simulink model "Feedforward"  (R2022a)
settings: Solver=VariableStepAuto  StartTime=0.0  StopTime=1000  RelTol=1e-3
undefined symbols (not defined in the file): C, k, k1, k2, k3, keta
libraries: slpidlib x1
settings Model: Creator=Anca Lombrea  LastModifiedBy=Anca Lombrea

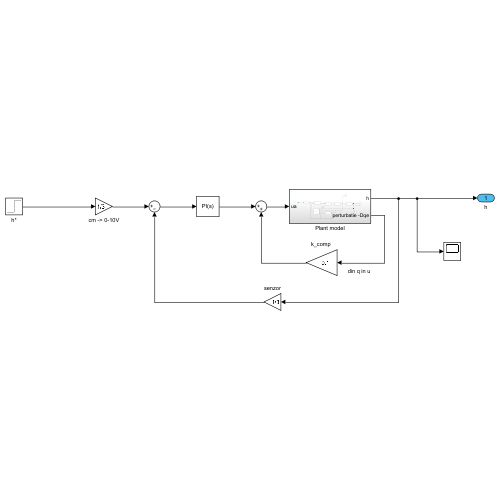
[thumbnail: Simulink's stored preview of the top-level diagram]
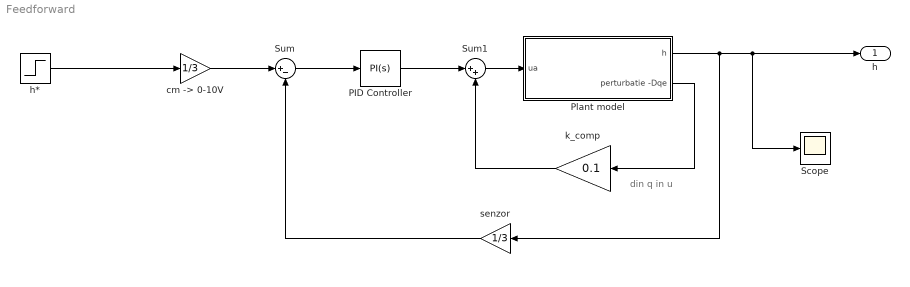
== system Feedforward ==
  note: din q in u
  PID Controller : slpidlib/PID Controller  Controller=PI  Form=Parallel  TimeDomain=Continuous-time  UseExternalTs=off  SampleTime=-1  IntegratorMethod=Forward Euler  FilterMethod=Forward Euler  ControllerParametersSource=internal  P=1.648  I=0.007925  UseKiTs=off  D=0  N=100  UseFilter=on  TunerSelectOption=Transfer Function Based (PID Tuner App)  InitialConditionSource=internal  InitialConditionForIntegrator=5.7  InitialConditionForFilter=0  DifferentiatorICPrevScaledInput=0  ExternalReset=none  TrackingMode=off  Kt=1  LimitOutput=off  SatLimitsSource=internal  UpperSaturationLimit=inf  LowerSaturationLimit=-inf  LinearizeAsGain=on  AntiWindupMode=none  Kb=1  POutMin=[]  POutMax=[]  IOutMin=[]  IOutMax=[]  DOutMin=[]  DOutMax=[]  NOutMin=[]  NOutMax=[]  SumOutMin=[]  SumOutMax=[]  SaturationOutMin=[]  SaturationOutMax=[]  PParamMin=[]  PParamMax=[]  IParamMin=[]  IParamMax=[]  DParamMin=[]  DParamMax=[]  NParamMin=[]  NParamMax=[]  KbParamMin=[]  KbParamMax=[]  KtParamMin=[]  KtParamMax=[]  KbOutMin=[]  KbOutMax=[]  KtOutMin=[]  KtOutMax=[]  IntegratorOutMin=[]  IntegratorOutMax=[]  FilterOutMin=[]  FilterOutMax=[]  SumI1OutMin=[]  SumI1OutMax=[]  SumI2OutMin=[]  SumI2OutMax=[]  SumI3OutMin=[]  SumI3OutMax=[]  SumI4OutMin=[]  SumI4OutMax=[]  SumDOutMin=[]  SumDOutMax=[]  DifferentiatorOutMin=[]  DifferentiatorOutMax=[]  FilterDiffOutCoefMin=[]  FilterDiffOutCoefMax=[]  ReciprocalOutMin=[]  ReciprocalOutMax=[]  SumDenOutMin=[]  SumDenOutMax=[]  SumNumOutMin=[]  SumNumOutMax=[]  DivideOutMin=[]  DivideOutMax=[]  UdiffTsProdOutMin=[]  UdiffTsProdOutMax=[]  NTsProdOutMin=[]  NTsProdOutMax=[]  UintegralTsProdOutMin=[]  UintegralTsProdOutMax=[]  UngainTsProdOutMin=[]  UngainTsProdOutMax=[]  IntegratorContinuousStateAttributes=''  IntegratorStateMustResolveToSignalObject=off  IntegratorRTWStateStorageClass=Auto  FilterContinuousStateAttributes=''  FilterStateMustResolveToSignalObject=off  FilterRTWStateStorageClass=Auto  ParallelPVariant=InternalParameters  IdealPVariant=Disabled  IVariant=InternalParameters  DVariant=Disabled  IntegratorVariant=Continuous  SatVariant=Disabled  AWVariant=Passthrough  PCopyVariant=Disabled  TRVariant=Disabled  FdbkBlocksVariant=Forward  IdealPFdbkVariant=Disabled  SatFdbkVariant=Disabled  DerivativeFilterVariant=Disabled  NVariant=Disabled  NCopyVariant=Disabled_SignalSpec  FilterICVariant=Disabled  IntegratorICVariant=InternalICs  ExternalResetVariant=Disabled  TRSumVariant=Passthrough  SumFdbkVariant=Disabled  SumVariant=Sum_PI  TsampFilterVariant=InternalTs  TsampNgainVariant=Passthrough  TsampIntegralVariant=Passthrough  ExternalSaturationOutDataTypeStr=Inherit: Same as second input  aMode=0
  Plant model : Subsystem
  Scope : Scope
  Sum : Sum  Inputs=|+-
  Sum1 : Sum  Inputs=|++
  "cm -> 0-10V" : Gain  Gain=1/3
  h* : Step  Time=0  After=20.87  SampleTime=0.01
  "k_comp " : Gain  Gain=0.1
  senzor : Gain  Gain=1/3
  h : Outport
  wires:
  senzor/1 -> Sum/2
  Sum/1 -> PID Controller/1
  Plant model/2(perturbatie -Dqe) -> "k_comp "/1
  h*/1 -> "cm -> 0-10V"/1
  Sum1/1 -> Plant model/1(ua)
  Plant model/1(h) -> senzor/1, Scope/1, h/1
  PID Controller/1 -> Sum1/1
  "cm -> 0-10V"/1 -> Sum/1
  "k_comp "/1 -> Sum1/2

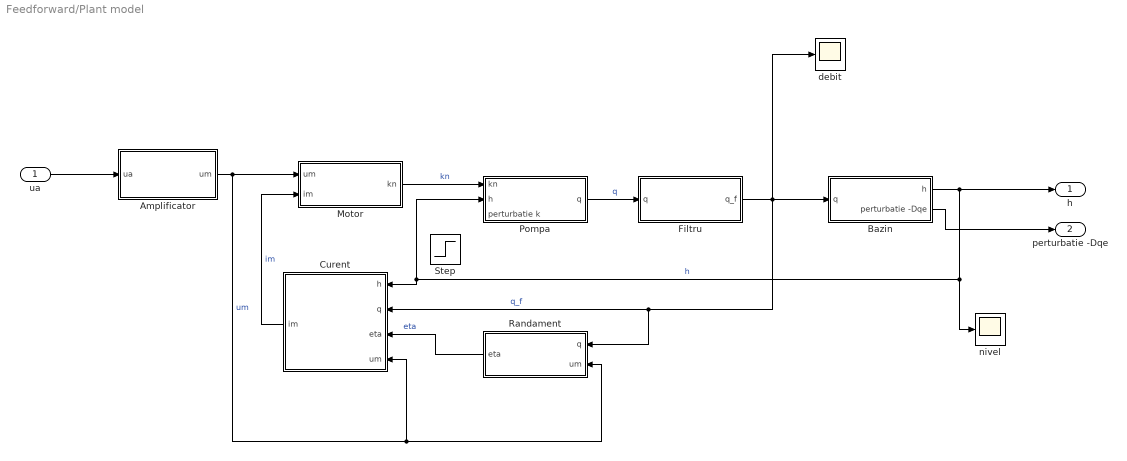
== system Feedforward/Plant model ==
  ua : Inport
  Amplificator : Subsystem
  Bazin : Subsystem
  Curent : Subsystem
  Filtru : Subsystem
  Motor : Subsystem
  Pompa : Subsystem
  Randament : Subsystem
  Step : Step  Time=250  Before=0.035  After=0.045  SampleTime=0
  debit : Scope
  nivel : Scope
  h : Outport
  perturbatie -Dqe : Outport  Port=2
  wires:
  Pompa/1("\tq") -> Filtru/1(q)  "q"
  Motor/1(kn) -> Pompa/1(kn)  "kn"
  Filtru/1(q_f) -> debit/1, Curent/2(q), Randament/1("\tq"), Bazin/1("\tq")  "q_f"
  ua/1 -> Amplificator/1(ua)
  Amplificator/1(um) -> Curent/4(um), Randament/2(um), Motor/1(um)  "um"
  Randament/1(eta) -> Curent/3(eta)  "eta"
  Bazin/1(h) -> nivel/1, Curent/1(h), Pompa/2(h), h/1  "h"
  Curent/1(im) -> Motor/2(im)  "im"
  Bazin/2(perturbatie -Dqe) -> perturbatie -Dqe/1

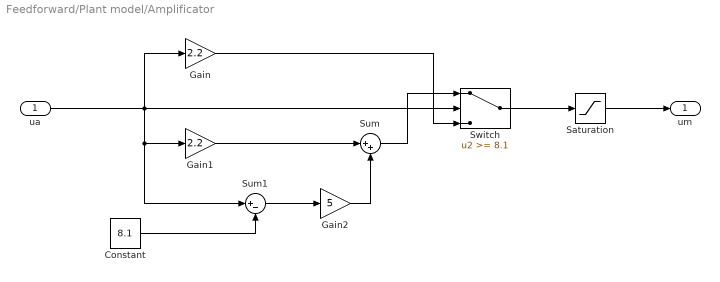
== system Feedforward/Plant model/Amplificator ==
  ua : Inport
  Constant : Constant  Value=8.1
  Gain : Gain  Gain=2.2
  Gain1 : Gain  Gain=2.2
  Gain2 : Gain  Gain=5
  Saturation : Saturate  UpperLimit=22  LowerLimit=0
  Sum : Sum  Inputs=|++
  Sum1 : Sum  Inputs=|+-
  Switch : Switch  Threshold=8.1  SaturateOnIntegerOverflow=off  InputSameDT=off
  um : Outport
  wires:
  Switch/1 -> Saturation/1
  Gain/1 -> Switch/3
  ua/1 -> Gain/1, Switch/2, Sum1/1, Gain1/1
  Gain2/1 -> Sum/2
  Constant/1 -> Sum1/2
  Sum/1 -> Switch/1
  Saturation/1 -> um/1
  Sum1/1 -> Gain2/1
  Gain1/1 -> Sum/1

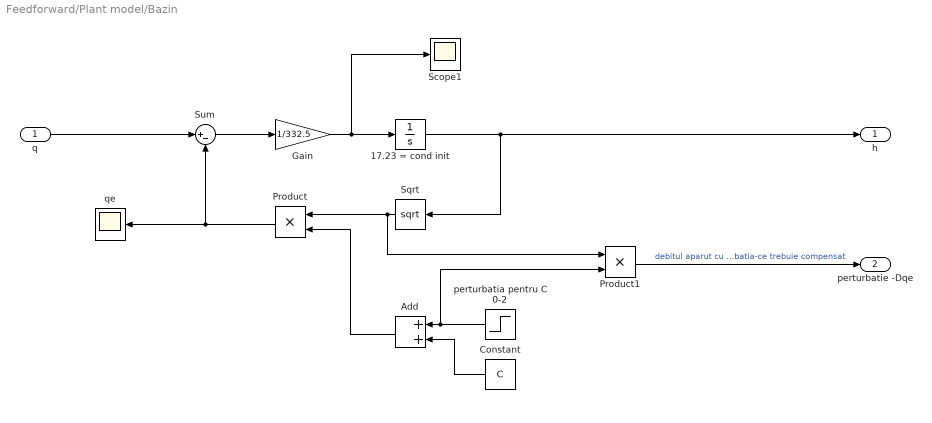
== system Feedforward/Plant model/Bazin ==
  "\tq" : Inport
  17.23 = cond init : Integrator  InitialCondition=17.23
  Add : Sum
  Constant : Constant  Value=C
  Gain : Gain  Gain=1/332.5
  Product : Product
  Product1 : Product
  Scope1 : Scope
  Sqrt : Sqrt
  Sum : Sum  Inputs=|+-
  "perturbatia pentru C 0-2 " : Step  Time=250  After=2  SampleTime=0
  qe : Scope
  h : Outport
  perturbatie -Dqe : Outport  Port=2
  wires:
  Sqrt/1 -> Product1/1, Product/1
  Product/1 -> qe/1, Sum/2
  "\tq"/1 -> Sum/1
  Sum/1 -> Gain/1
  17.23 = cond init/1 -> Sqrt/1, h/1
  Gain/1 -> 17.23 = cond init/1, Scope1/1
  "perturbatia pentru C 0-2 "/1 -> Product1/2, Add/1
  Constant/1 -> Add/2
  Add/1 -> Product/2
  Product1/1 -> perturbatie -Dqe/1  "debitul aparut cu perturbatia-ce trebuie compensat"

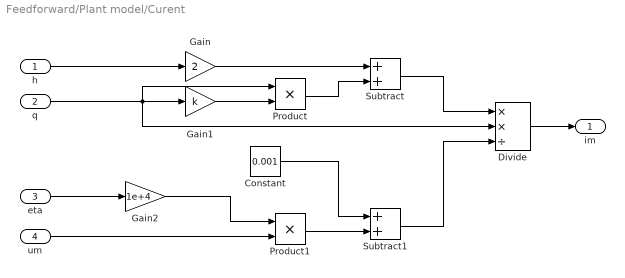
== system Feedforward/Plant model/Curent ==
  h : Inport
  q : Inport  Port=2
  eta : Inport  Port=3
  um : Inport  Port=4
  Constant : Constant  Value=0.001
  Divide : Product  Inputs=**/
  Gain : Gain  Gain=2
  Gain1 : Gain  Gain=k
  Gain2 : Gain  Gain=1e+4
  Product : Product
  Product1 : Product
  Subtract : Sum
  Subtract1 : Sum
  im : Outport
  wires:
  h/1 -> Gain/1
  Gain/1 -> Subtract/1
  q/1 -> Divide/2, Gain1/1, Product/1
  Gain1/1 -> Product/2
  Product/1 -> Subtract/2
  Subtract/1 -> Divide/1
  eta/1 -> Gain2/1
  Gain2/1 -> Product1/1
  um/1 -> Product1/2
  Product1/1 -> Subtract1/2
  Constant/1 -> Subtract1/1
  Subtract1/1 -> Divide/3
  Divide/1 -> im/1

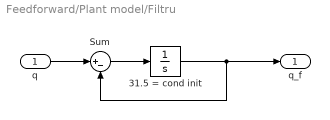
== system Feedforward/Plant model/Filtru ==
  q : Inport
  31.5 = cond init : Integrator  InitialCondition=31.5
  Sum : Sum  Inputs=|+-
  q_f : Outport
  wires:
  31.5 = cond init/1 -> Sum/2, q_f/1
  q/1 -> Sum/1
  Sum/1 -> 31.5 = cond init/1

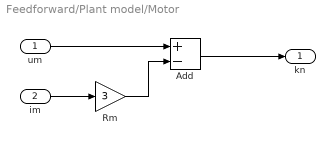
== system Feedforward/Plant model/Motor ==
  um : Inport
  im : Inport  Port=2
  Add : Sum  Inputs=+-
  Rm : Gain  Gain=3
  kn : Outport
  wires:
  im/1 -> Rm/1
  Rm/1 -> Add/2
  um/1 -> Add/1
  Add/1 -> kn/1

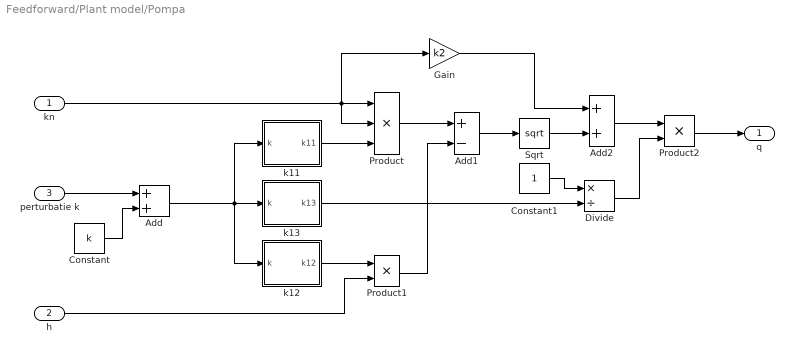
== system Feedforward/Plant model/Pompa ==
  kn : Inport
  h : Inport  Port=2
  perturbatie k : Inport  Port=3
  Add : Sum
  Add1 : Sum  Inputs=+-
  Add2 : Sum
  Constant : Constant  Value=k
  Constant1 : Constant
  Divide : Product  Inputs=*/
  Gain : Gain  Gain=k2
  Product : Product  Inputs=3
  Product1 : Product
  Product2 : Product
  Sqrt : Sqrt
  k11 : Subsystem
  k12 : Subsystem
  k13 : Subsystem
  "\tq" : Outport
  wires:
  perturbatie k/1 -> Add/1
  Constant/1 -> Add/2
  Add/1 -> k12/1(k), k13/1(k), k11/1(k)
  k11/1(k11) -> Product/3
  kn/1 -> Gain/1, Product/2, Product/1
  Product/1 -> Add1/1
  h/1 -> Product1/2
  k12/1(k12) -> Product1/1
  Product1/1 -> Add1/2
  Add1/1 -> Sqrt/1
  Sqrt/1 -> Add2/2
  Gain/1 -> Add2/1
  k13/1(k13) -> Divide/2
  Constant1/1 -> Divide/1
  Add2/1 -> Product2/1
  Divide/1 -> Product2/2
  Product2/1 -> "\tq"/1

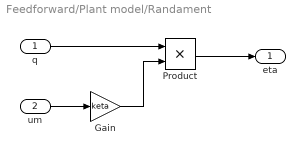
== system Feedforward/Plant model/Randament ==
  "\tq" : Inport
  um : Inport  Port=2
  Gain : Gain  Gain=keta
  Product : Product
  eta : Outport
  wires:
  um/1 -> Gain/1
  "\tq"/1 -> Product/1
  Gain/1 -> Product/2
  Product/1 -> eta/1

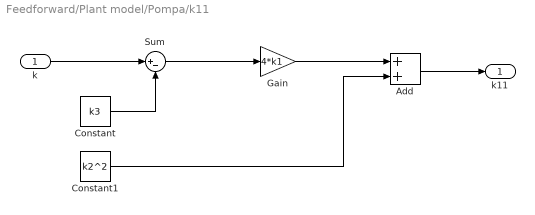
== system Feedforward/Plant model/Pompa/k11 ==
  k : Inport
  Add : Sum
  Constant : Constant  Value=k3
  Constant1 : Constant  Value=k2^2
  Gain : Gain  Gain=4*k1
  Sum : Sum  Inputs=|+-
  k11 : Outport
  wires:
  Add/1 -> k11/1
  k/1 -> Sum/1
  Constant/1 -> Sum/2
  Sum/1 -> Gain/1
  Gain/1 -> Add/1
  Constant1/1 -> Add/2

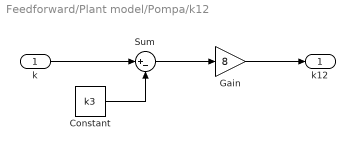
== system Feedforward/Plant model/Pompa/k12 ==
  k : Inport
  Constant : Constant  Value=k3
  Gain : Gain  Gain=8
  Sum : Sum  Inputs=|+-
  k12 : Outport
  wires:
  k/1 -> Sum/1
  Constant/1 -> Sum/2
  Sum/1 -> Gain/1
  Gain/1 -> k12/1

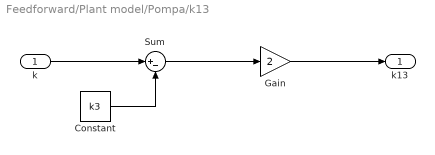
== system Feedforward/Plant model/Pompa/k13 ==
  k : Inport
  Constant : Constant  Value=k3
  Gain : Gain  Gain=2
  Sum : Sum  Inputs=|+-
  k13 : Outport
  wires:
  k/1 -> Sum/1
  Constant/1 -> Sum/2
  Gain/1 -> k13/1
  Sum/1 -> Gain/1
